simulink model "model"  (R2018b)
settings: Solver=FixedStepAuto  StartTime=0.0  StopTime=Np*Ts  FixedStep=Ts  RelTol=1e-3
values from neighbouring files (symbols this model uses):
  A = [0 1;-1 -2]    [test.m]
  Ad = (eye(2)+Ts*A/2)/((eye(2)-Ts*A/2))    [test.m]
  B = [0 1]'    [test.m]
  Bd = Ts*B    [test.m]
  C = [1 0]    [test.m]
  Cd = C    [test.m]
  D = 0    [test.m]
  Dd = D    (= 0)    [test.m]
  Ts = 0.1    [test.m]
  X0 = [1 2]'    [test.m]
settings Model: Creator=le'e'x'  LastModifiedBy=le'e'x'

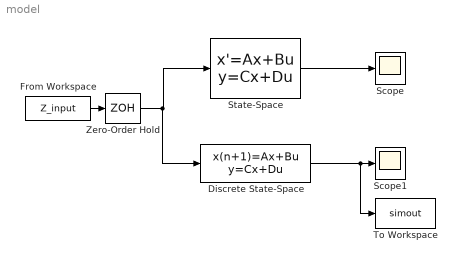
== system model ==
  Discrete State-Space : DiscreteStateSpace  A=Ad  B=Bd  C=Cd  D=Dd  InitialCondition=X0  SampleTime=Ts
  From Workspace : FromWorkspace  VariableName=Z_input  SampleTime=0
  Scope : Scope
  Scope1 : Scope
  State-Space : StateSpace  A=A  B=B  C=C  D=D  InitialCondition=X0
  To Workspace : ToWorkspace  VariableName=simout  SaveFormat=Structure With Time  SampleTime=-1
  Zero-Order Hold : ZeroOrderHold  SampleTime=-1
  wires:
  Zero-Order Hold/1 -> Discrete State-Space/1, State-Space/1
  State-Space/1 -> Scope/1
  Discrete State-Space/1 -> To Workspace/1, Scope1/1
  From Workspace/1 -> Zero-Order Hold/1
